simulink model "untitled"  (Simulink 8.5)
settings: Solver=ode45  StartTime=0.0  StopTime=0.04  FixedStep=0.0001  RelTol=1e-3
libraries: powerlib x131
settings Model: Creator=yahya  LastModifiedBy=yahya
settings DebuggingCC: SolverPrmCheckMsg=warning  FcnCallInpInsideContextMsg=EnableAllAsWarning
settings GRTTargetCC: CombineOutputUpdateFcns=on  GRTInterface=off

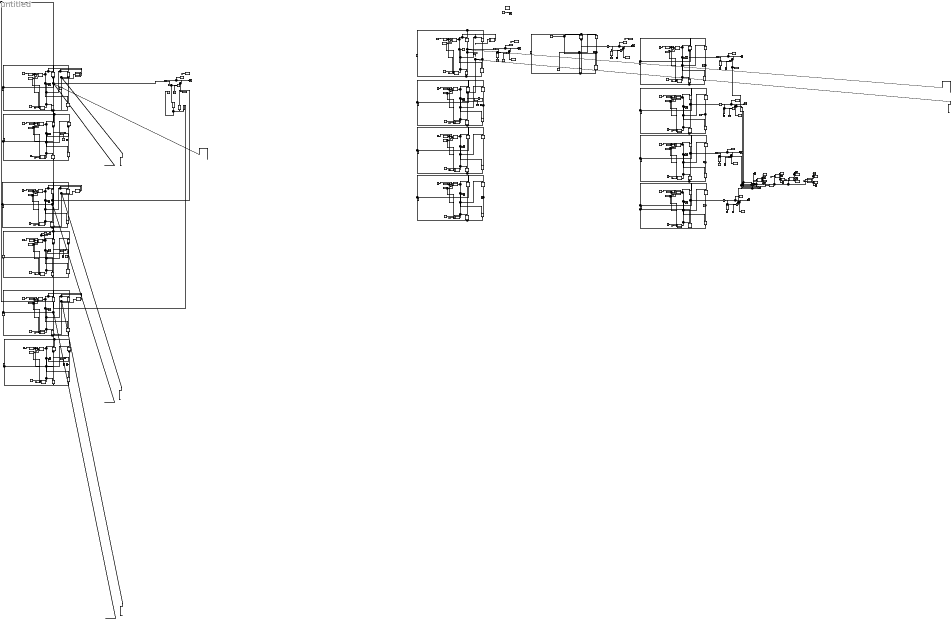
== system untitled ==
  Clock{,1..34} (35 alike) : Clock
  Current Measurement{,1..6} (7 alike) : powerlib/Measurements/Current Measurement  PhasorSimulation=off  OutputType=Complex  PSBequivalent=0
  DC Voltage Source{,1..14} (15 alike) : powerlib/Electrical Sources/DC Voltage Source  Amplitude=100  Measurements=None
  From Workspace1 : FromWorkspace  VariableName=tetha12  SampleTime=0
  From Workspace10 : FromWorkspace  VariableName=tetha11  SampleTime=0
  From Workspace{2,4,6,8,11..12,14,16,18,20,22,24,26,33} (14 alike) : FromWorkspace  VariableName=fs  SampleTime=0
  From Workspace13 : FromWorkspace  VariableName=tetha14  SampleTime=0
  From Workspace15 : FromWorkspace  VariableName=tetha12  SampleTime=0
  From Workspace17 : FromWorkspace  VariableName=tetha11  SampleTime=0
  From Workspace19 : FromWorkspace  VariableName=tetha12_120  SampleTime=0
  From Workspace21 : FromWorkspace  VariableName=tetha11_120  SampleTime=0
  From Workspace23 : FromWorkspace  VariableName=tetha12_240  SampleTime=0
  From Workspace25 : FromWorkspace  VariableName=tetha11_240  SampleTime=0
  From Workspace3 : FromWorkspace  VariableName=tetha13  SampleTime=0
  From Workspace32 : FromWorkspace  VariableName=tetha11  SampleTime=0
  From Workspace5 : FromWorkspace  VariableName=tetha14  SampleTime=0
  From Workspace7 : FromWorkspace  VariableName=tetha12  SampleTime=0
  From Workspace9 : FromWorkspace  VariableName=tetha13  SampleTime=0
  Ground{1..28} (28 alike) : powerlib/Elements/Ground  LConnTagsString=a
  IGBT/Diode{1..60} (60 alike) : powerlib/Power Electronics/IGBT//Diode  Ron=1e-3  Rs=1e5  Cs=inf  Measurements=off
  MATLAB Function : MATLAB Function  TreatAsAtomicUnit=on
  MATLAB Function1 : MATLAB Function  TreatAsAtomicUnit=on
  MATLAB Function10 : MATLAB Function  TreatAsAtomicUnit=on
  MATLAB Function11 : MATLAB Function  TreatAsAtomicUnit=on
  MATLAB Function12 : MATLAB Function  TreatAsAtomicUnit=on
  MATLAB Function13 : MATLAB Function  TreatAsAtomicUnit=on
  MATLAB Function14 : MATLAB Function  TreatAsAtomicUnit=on
  MATLAB Function15 : MATLAB Function  TreatAsAtomicUnit=on
  MATLAB Function16 : MATLAB Function  TreatAsAtomicUnit=on
  MATLAB Function17 : MATLAB Function  TreatAsAtomicUnit=on
  MATLAB Function18 : MATLAB Function  TreatAsAtomicUnit=on
  MATLAB Function19 : MATLAB Function  TreatAsAtomicUnit=on
  MATLAB Function2 : MATLAB Function  TreatAsAtomicUnit=on
  MATLAB Function20 : MATLAB Function  TreatAsAtomicUnit=on
  MATLAB Function21 : MATLAB Function  TreatAsAtomicUnit=on
  MATLAB Function22 : MATLAB Function  TreatAsAtomicUnit=on
  MATLAB Function23 : MATLAB Function  TreatAsAtomicUnit=on
  MATLAB Function24 : MATLAB Function  TreatAsAtomicUnit=on
  MATLAB Function25 : MATLAB Function  TreatAsAtomicUnit=on
  MATLAB Function26 : MATLAB Function  TreatAsAtomicUnit=on
  MATLAB Function27 : MATLAB Function  TreatAsAtomicUnit=on
  MATLAB Function28 : MATLAB Function  TreatAsAtomicUnit=on
  MATLAB Function29 : MATLAB Function  TreatAsAtomicUnit=on
  MATLAB Function3 : MATLAB Function  TreatAsAtomicUnit=on
  MATLAB Function30 : MATLAB Function  TreatAsAtomicUnit=on
  MATLAB Function31 : MATLAB Function  TreatAsAtomicUnit=on
  MATLAB Function32 : MATLAB Function  TreatAsAtomicUnit=on
  MATLAB Function33 : MATLAB Function  TreatAsAtomicUnit=on
  MATLAB Function34 : MATLAB Function  TreatAsAtomicUnit=on
  MATLAB Function35 : MATLAB Function  TreatAsAtomicUnit=on
  MATLAB Function4 : MATLAB Function  TreatAsAtomicUnit=on
  MATLAB Function5 : MATLAB Function  TreatAsAtomicUnit=on
  MATLAB Function6 : MATLAB Function  TreatAsAtomicUnit=on
  MATLAB Function7 : MATLAB Function  TreatAsAtomicUnit=on
  MATLAB Function8 : MATLAB Function  TreatAsAtomicUnit=on
  MATLAB Function9 : MATLAB Function  TreatAsAtomicUnit=on
  Pulse Generator{,2,5,7..8,11,13,15,17,19,21} (11 alike) : DiscretePulseGenerator  PulseType=Time based  Amplitude=10  Period=0.02  PulseWidth=50
  Pulse Generator{1,3,6,9..10,12,14,16,18,20,22} (11 alike) : DiscretePulseGenerator  PulseType=Time based  Amplitude=10  Period=0.02  PulseWidth=50  PhaseDelay=0.01
  Pulse Generator23 : DiscretePulseGenerator  PulseType=Time based  Amplitude=10  Period=0.02  PulseWidth=50  PhaseDelay=0.006666666666667
  Pulse Generator24 : DiscretePulseGenerator  PulseType=Time based  Amplitude=10  Period=0.02  PulseWidth=50  PhaseDelay=0.01+0.006666666666667
  Pulse Generator25 : DiscretePulseGenerator  PulseType=Time based  Amplitude=10  Period=0.02  PulseWidth=50  PhaseDelay=0.006666666666667
  Pulse Generator26 : DiscretePulseGenerator  PulseType=Time based  Amplitude=10  Period=0.02  PulseWidth=50  PhaseDelay=0.01+0.006666666666667
  Pulse Generator27 : DiscretePulseGenerator  PulseType=Time based  Amplitude=10  Period=0.02  PulseWidth=50  PhaseDelay=2*0.006666666666667
  Pulse Generator28 : DiscretePulseGenerator  PulseType=Time based  Amplitude=10  Period=0.02  PulseWidth=50  PhaseDelay=0.01+2*0.006666666666667
  Pulse Generator29 : DiscretePulseGenerator  PulseType=Time based  Amplitude=10  Period=0.02  PulseWidth=50  PhaseDelay=2*0.006666666666667
  Pulse Generator30 : DiscretePulseGenerator  PulseType=Time based  Amplitude=10  Period=0.02  PulseWidth=50  PhaseDelay=0.01+2*0.006666666666667
  Pulse Generator4 : DiscretePulseGenerator  PulseType=Time based  Period=0.0001  PulseWidth=50
  Scope{,1,4,6..14,25} (13 alike) : Scope  NumInputPorts=2
      Scope settings: TimeRange=1  YMin=-400~-400  YMax=400~400
      Scope1 settings: TimeRange=1  YMin=-400~-400  YMax=400~400
      Scope10 settings: TimeRange=1  YMin=-400~-400  YMax=400~400  SaveName=ScopeData4
      Scope11 settings: TimeRange=1  YMin=-400~-400  YMax=400~400  SaveName=ScopeData11
      Scope12 settings: TimeRange=1  YMin=-400~-400  YMax=400~400  SaveName=ScopeData12
      Scope13 settings: TimeRange=1  YMin=-400~-400  YMax=400~400  SaveName=ScopeData13
      Scope14 settings: TimeRange=1  YMin=-400~-400  YMax=400~400  SaveName=ScopeData14
      Scope25 settings: TimeRange=1  YMin=-400~-400  YMax=400~400  SaveName=ScopeData25
      Scope4 settings: TimeRange=1  YMin=-400~-400  YMax=400~400  SaveName=ScopeData6
      Scope6 settings: TimeRange=1  YMin=-400~-400  YMax=400~400  SaveName=ScopeData7
      Scope7 settings: TimeRange=1  YMin=-400~-400  YMax=400~400  SaveName=ScopeData9
      Scope8 settings: TimeRange=1  YMin=-400~-400  YMax=400~400  SaveName=ScopeData8
      Scope9 settings: TimeRange=1  YMin=-400~-400  YMax=400~400  SaveName=ScopeData10
  Scope15 : Scope  NumInputPorts=4
      settings: TimeRange=1  YMin=-400~-400~-5~-5  YMax=400~400~5~5  SaveName=ScopeData15
  Scope{16..24} (9 alike) : Scope
      Scope16 settings: TimeRange=0.2  YMin=190  YMax=400  SaveName=ScopeData16
      Scope17 settings: TimeRange=0.2  YMin=190  YMax=400  SaveName=ScopeData17
      Scope18 settings: TimeRange=0.2  YMin=190  YMax=400  SaveName=ScopeData18
      Scope19 settings: TimeRange=0.2  YMin=190  YMax=400  SaveName=ScopeData19
      Scope20 settings: TimeRange=0.2  YMin=190  YMax=400  SaveName=ScopeData20
      Scope21 settings: TimeRange=0.2  YMin=190  YMax=400  SaveName=ScopeData21
      Scope22 settings: TimeRange=0.2  YMin=190  YMax=400  SaveName=ScopeData22
      Scope23 settings: TimeRange=0.2  YMin=190  YMax=400  SaveName=ScopeData23
      Scope24 settings: TimeRange=0.2  YMin=190  YMax=400  SaveName=ScopeData24
  Scope{2..3,5,26..32} (10 alike) : Scope  NumInputPorts=3
      Scope2 settings: TimeRange=1  YMin=-400~-400~-5  YMax=400~400~5  SaveName=ScopeData3
      Scope26 settings: TimeRange=1  YMin=-400~-400~-5  YMax=400~400~5  SaveName=ScopeData26
      Scope27 settings: TimeRange=1  YMin=-400~-400~-5  YMax=400~400~5  SaveName=ScopeData27
      Scope28 settings: TimeRange=1  YMin=-400~-400~-5  YMax=400~400~5  SaveName=ScopeData28
      Scope29 settings: TimeRange=1  YMin=-400~-400~-5  YMax=400~400~5  SaveName=ScopeData29
      Scope3 settings: TimeRange=0.03572500664993174  YMin=-1~0~0  YMax=1~10~10  SaveName=ScopeData2
      Scope30 settings: TimeRange=1  YMin=-400~-400~-5  YMax=400~400~5  SaveName=ScopeData30
      Scope31 settings: TimeRange=1  YMin=-400~-400~-5  YMax=400~400~5  SaveName=ScopeData31
      Scope32 settings: TimeRange=1  YMin=-400~-400~-5  YMax=400~400~5  SaveName=ScopeData32
      Scope5 settings: TimeRange=1  YMin=-400~-400~-5  YMax=400~400~5  SaveName=ScopeData5
  Series RLC Branch{,6..8} (4 alike) : powerlib/Elements/Series RLC Branch  LConnTagsString=__new0  RConnTagsString=__new0  BranchType=R  Resistance=1  Inductance=1e-3  SetiL0=off  InitialCurrent=0  Capacitance=1e-6  Setx0=off  InitialVoltage=0  Measurements=None
  Series RLC Branch1 : powerlib/Elements/Series RLC Branch  LConnTagsString=__new0  RConnTagsString=__new0  BranchType=RL  Resistance=1  Inductance=1e-3  SetiL0=off  InitialCurrent=0  Capacitance=1e-6  Setx0=off  InitialVoltage=0  Measurements=None
  Series RLC Branch{2..5} (4 alike) : powerlib/Elements/Series RLC Branch  LConnTagsString=__new0  RConnTagsString=__new0  BranchType=R  Resistance=1  Inductance=1e-5  SetiL0=off  InitialCurrent=0  Capacitance=1e-6  Setx0=off  InitialVoltage=0  Measurements=None
  Sum : Sum  Inputs=|++++
  To Workspace : ToWorkspace  VariableName=i  SaveFormat=Timeseries  SampleTime=-1
  To Workspace1 : ToWorkspace  VariableName=v  SaveFormat=Timeseries  SampleTime=-1
  To Workspace10 : ToWorkspace  VariableName=v3  SaveFormat=Timeseries  SampleTime=-1
  To Workspace11 : ToWorkspace  VariableName=A1  SaveFormat=Timeseries  SampleTime=-1
  To Workspace12 : ToWorkspace  VariableName=i4  SaveFormat=Timeseries  SampleTime=-1
  To Workspace13 : ToWorkspace  VariableName=v4  SaveFormat=Timeseries  SampleTime=-1
  To Workspace14 : ToWorkspace  VariableName=B1  SaveFormat=Timeseries  SampleTime=-1
  To Workspace15 : ToWorkspace  VariableName=i5  SaveFormat=Timeseries  SampleTime=-1
  To Workspace16 : ToWorkspace  VariableName=v5  SaveFormat=Timeseries  SampleTime=-1
  To Workspace17 : ToWorkspace  VariableName=A7  SaveFormat=Timeseries  SampleTime=-1
  To Workspace18 : ToWorkspace  VariableName=B7  SaveFormat=Timeseries  SampleTime=-1
  To Workspace19 : ToWorkspace  VariableName=A11  SaveFormat=Timeseries  SampleTime=-1
  To Workspace2 : ToWorkspace  VariableName=t  SaveFormat=Timeseries  SampleTime=-1
  To Workspace20 : ToWorkspace  VariableName=B11  SaveFormat=Timeseries  SampleTime=-1
  To Workspace21 : ToWorkspace  VariableName=A5  SaveFormat=Timeseries  SampleTime=-1
  To Workspace22 : ToWorkspace  VariableName=B5  SaveFormat=Timeseries  SampleTime=-1
  To Workspace23 : ToWorkspace  VariableName=i6  SaveFormat=Timeseries  SampleTime=-1
  To Workspace24 : ToWorkspace  VariableName=v6  SaveFormat=Timeseries  SampleTime=-1
  To Workspace25 : ToWorkspace  VariableName=t2  SaveFormat=Timeseries  SampleTime=-1
  To Workspace3 : ToWorkspace  VariableName=i1  SaveFormat=Timeseries  SampleTime=-1
  To Workspace4 : ToWorkspace  VariableName=v1  SaveFormat=Timeseries  SampleTime=-1
  To Workspace5 : ToWorkspace  VariableName=t1  SaveFormat=Timeseries  SampleTime=-1
  To Workspace6 : ToWorkspace  VariableName=i2  SaveFormat=Timeseries  SampleTime=-1
  To Workspace7 : ToWorkspace  VariableName=v2  SaveFormat=Timeseries  SampleTime=-1
  To Workspace8 : ToWorkspace  VariableName=v_phase  SaveFormat=Timeseries  SampleTime=-1
  To Workspace9 : ToWorkspace  VariableName=i3  SaveFormat=Timeseries  SampleTime=-1
  Unit Delay : UnitDelay  SampleTime=0.01
  Voltage Measurement{,1..10} (11 alike) : powerlib/Measurements/Voltage Measurement  PhasorSimulation=off  OutputType=Complex  PSBequivalent=0
  powergui : powerlib/powergui  Priority=1  SimulationMode=Continuous  SolverType=Tustin/Backward Euler (TBE)  SampleTime=50e-6  frequency=60  SPID=off  DisableSnubberDevices=off  DisableRonSwitches=off  DisableVfSwitches=off  SwTol=0  DisplayEquations=off  Interpol=off  methode=off  Ts=100  FunctionMessages=off  echomessages=off  HookPort=off  EnableUseOfTLC=off  x0status=blocks  frequencyindice=0  Pbase=100e6  ErrMax=1e-4  Iterations=50  UnitsV=kV  UnitsW=MW  buscounter=0  RestoreLinks=warning  ResistiveCurrentMeasurement=off  Frange=[0:2:500]  Ylog=off  Xlog=on  ShowGrid=off  save=off  variable=ZData  structure=0  ZoomFFT=off  StartTime=0.0  cycles=1  DisplayStyle=1  fundamental=60  FreqAxis=off  MaxFrequency=1000  frequencyindicesteady=1  RmsSteady=1  display=off
  wires:
  Current Measurement/1 -> To Workspace/1, Scope/1
  Voltage Measurement/1 -> To Workspace1/1, Scope/2
  Clock/1 -> To Workspace2/1
  From Workspace32/1 -> MATLAB Function1/2(t), MATLAB Function/2(t)
  From Workspace33/1 -> MATLAB Function1/4(fs), MATLAB Function/4(fs)
  Clock1/1 -> MATLAB Function/3(time)
  Pulse Generator/1 -> MATLAB Function/1(u)
  Clock2/1 -> MATLAB Function1/3(time)
  Pulse Generator1/1 -> MATLAB Function1/1(u)
  Current Measurement1/1 -> To Workspace3/1, Scope1/1
  Voltage Measurement1/1 -> To Workspace4/1, Scope1/2
  Clock3/1 -> To Workspace5/1
  Pulse Generator3/1 -> IGBT/Diode6/1, IGBT/Diode7/1
  Pulse Generator2/1 -> IGBT/Diode8/1, IGBT/Diode5/1
  Pulse Generator4/1 -> Scope3/1
  MATLAB Function/1(y) -> MATLAB Function20/1(u1), IGBT/Diode1/1, IGBT/Diode4/1, Scope2/1
  MATLAB Function1/1(y) -> IGBT/Diode3/1, MATLAB Function20/2(u2), IGBT/Diode2/1, Scope2/2
  From Workspace1/1 -> MATLAB Function3/2(t), MATLAB Function2/2(t)
  From Workspace2/1 -> MATLAB Function3/4(fs), MATLAB Function2/4(fs)
  Clock5/1 -> MATLAB Function2/3(time)
  Pulse Generator5/1 -> MATLAB Function2/1(u)
  Clock6/1 -> MATLAB Function3/3(time)
  Pulse Generator6/1 -> MATLAB Function3/1(u)
  MATLAB Function2/1(y) -> IGBT/Diode9/1, IGBT/Diode12/1, Scope5/1
  MATLAB Function3/1(y) -> IGBT/Diode11/1, IGBT/Diode10/1, Scope5/2
  From Workspace3/1 -> MATLAB Function5/2(t), MATLAB Function4/2(t)
  From Workspace4/1 -> MATLAB Function5/4(fs), MATLAB Function4/4(fs)
  Clock8/1 -> MATLAB Function4/3(time)
  Pulse Generator8/1 -> MATLAB Function4/1(u)
  Clock9/1 -> MATLAB Function5/3(time)
  Pulse Generator9/1 -> MATLAB Function5/1(u)
  MATLAB Function4/1(y) -> IGBT/Diode13/1, IGBT/Diode16/1, Scope8/1
  MATLAB Function5/1(y) -> IGBT/Diode15/1, IGBT/Diode14/1, Scope8/2
  From Workspace5/1 -> MATLAB Function7/2(t), MATLAB Function6/2(t)
  From Workspace6/1 -> MATLAB Function7/4(fs), MATLAB Function6/4(fs)
  Clock11/1 -> MATLAB Function6/3(time)
  Pulse Generator11/1 -> MATLAB Function6/1(u)
  Clock12/1 -> MATLAB Function7/3(time)
  Pulse Generator12/1 -> MATLAB Function7/1(u)
  MATLAB Function6/1(y) -> IGBT/Diode17/1, IGBT/Diode20/1, Scope11/1
  MATLAB Function7/1(y) -> IGBT/Diode19/1, IGBT/Diode18/1, Scope11/2
  Current Measurement2/1 -> To Workspace6/1, Scope4/1
  Voltage Measurement2/1 -> Sum/1, Scope15/1, To Workspace7/1, Scope4/2
  From Workspace10/1 -> MATLAB Function9/2(t), MATLAB Function8/2(t)
  From Workspace11/1 -> MATLAB Function9/4(fs), MATLAB Function8/4(fs)
  Clock7/1 -> MATLAB Function8/3(time)
  Pulse Generator7/1 -> MATLAB Function8/1(u)
  Clock14/1 -> MATLAB Function9/3(time)
  Pulse Generator10/1 -> MATLAB Function9/1(u)
  MATLAB Function8/1(y) -> IGBT/Diode21/1, IGBT/Diode35/1, Scope7/1
  MATLAB Function9/1(y) -> IGBT/Diode34/1, IGBT/Diode32/1, Scope7/2
  From Workspace7/1 -> MATLAB Function11/2(t), MATLAB Function10/2(t)
  From Workspace8/1 -> MATLAB Function11/4(fs), MATLAB Function10/4(fs)
  Clock15/1 -> MATLAB Function10/3(time)
  Pulse Generator15/1 -> MATLAB Function10/1(u)
  Clock16/1 -> MATLAB Function11/3(time)
  Pulse Generator16/1 -> MATLAB Function11/1(u)
  MATLAB Function10/1(y) -> IGBT/Diode36/1, IGBT/Diode24/1, Scope9/1
  MATLAB Function11/1(y) -> IGBT/Diode23/1, IGBT/Diode22/1, Scope9/2
  From Workspace9/1 -> MATLAB Function13/2(t), MATLAB Function12/2(t)
  From Workspace12/1 -> MATLAB Function13/4(fs), MATLAB Function12/4(fs)
  Clock17/1 -> MATLAB Function12/3(time)
  Pulse Generator17/1 -> MATLAB Function12/1(u)
  Clock18/1 -> MATLAB Function13/3(time)
  Pulse Generator18/1 -> MATLAB Function13/1(u)
  MATLAB Function12/1(y) -> IGBT/Diode25/1, IGBT/Diode28/1, Scope10/1
  MATLAB Function13/1(y) -> IGBT/Diode27/1, IGBT/Diode26/1, Scope10/2
  From Workspace13/1 -> MATLAB Function15/2(t), MATLAB Function14/2(t)
  From Workspace14/1 -> MATLAB Function15/4(fs), MATLAB Function14/4(fs)
  Clock10/1 -> MATLAB Function14/3(time)
  Pulse Generator13/1 -> MATLAB Function14/1(u)
  Clock13/1 -> MATLAB Function15/3(time)
  Pulse Generator14/1 -> MATLAB Function15/1(u)
  MATLAB Function14/1(y) -> IGBT/Diode29/1, IGBT/Diode33/1, Scope6/1
  MATLAB Function15/1(y) -> IGBT/Diode31/1, IGBT/Diode30/1, Scope6/2
  Current Measurement3/1 -> To Workspace9/1, Scope12/1
  Voltage Measurement3/1 -> Sum/2, Scope15/2, Scope12/2, To Workspace10/1
  Current Measurement4/1 -> To Workspace12/1, Scope13/1
  Voltage Measurement4/1 -> Scope15/3, Sum/3, To Workspace13/1, Scope13/2
  Current Measurement5/1 -> To Workspace15/1, Scope14/1
  Voltage Measurement5/1 -> Sum/4, Scope15/4, To Workspace16/1, Scope14/2
  Clock4/1 -> MATLAB Function16/2(time)
  MATLAB Function16/1(A1) -> To Workspace11/1, Scope17/1
  MATLAB Function16/2(B1) -> Scope18/1, To Workspace14/1
  Clock19/1 -> MATLAB Function17/2(time)
  MATLAB Function17/1(A7) -> Scope16/1, To Workspace17/1
  MATLAB Function17/2(B7) -> To Workspace18/1, Scope19/1
  Sum/1 -> Scope24/1, MATLAB Function18/1(u), MATLAB Function17/1(u), MATLAB Function19/1(u), To Workspace8/1, MATLAB Function16/1(u)
  Clock20/1 -> MATLAB Function18/2(time)
  MATLAB Function18/1(A11) -> Scope20/1, To Workspace19/1
  MATLAB Function18/2(B11) -> Scope21/1, To Workspace20/1
  Clock21/1 -> MATLAB Function19/2(time)
  MATLAB Function19/1(A5) -> Scope22/1, To Workspace21/1
  MATLAB Function19/2(B5) -> Scope23/1, To Workspace22/1
  ? -> Scope2/3
  Voltage Measurement7/1 -> Scope5/3
  MATLAB Function20/1(y) -> ?
  Current Measurement6/1 -> Scope25/1, To Workspace23/1
  Voltage Measurement6/1 -> To Workspace24/1, Scope25/2
  Clock22/1 -> To Workspace25/1
  From Workspace17/1 -> MATLAB Function22/2(t), MATLAB Function21/2(t)
  From Workspace18/1 -> MATLAB Function22/4(fs), MATLAB Function21/4(fs)
  Clock23/1 -> MATLAB Function21/3(time)
  Pulse Generator19/1 -> MATLAB Function21/1(u)
  Clock24/1 -> MATLAB Function22/3(time)
  Pulse Generator20/1 -> MATLAB Function22/1(u)
  MATLAB Function21/1(y) -> MATLAB Function24/1(u1), IGBT/Diode37/1, IGBT/Diode43/1, Scope26/1
  MATLAB Function22/1(y) -> IGBT/Diode42/1, MATLAB Function24/2(u2), IGBT/Diode41/1, Scope26/2
  From Workspace15/1 -> MATLAB Function25/2(t), MATLAB Function23/2(t)
  From Workspace16/1 -> MATLAB Function25/4(fs), MATLAB Function23/4(fs)
  Clock25/1 -> MATLAB Function23/3(time)
  Pulse Generator21/1 -> MATLAB Function23/1(u)
  Clock26/1 -> MATLAB Function25/3(time)
  Pulse Generator22/1 -> MATLAB Function25/1(u)
  MATLAB Function23/1(y) -> IGBT/Diode44/1, IGBT/Diode40/1, Scope27/1
  MATLAB Function25/1(y) -> IGBT/Diode39/1, IGBT/Diode38/1, Scope27/2
  ? -> Scope26/3
  Voltage Measurement8/1 -> Scope27/3
  MATLAB Function24/1(y) -> ?
  From Workspace21/1 -> MATLAB Function27/2(t), MATLAB Function26/2(t)
  From Workspace22/1 -> MATLAB Function27/4(fs), MATLAB Function26/4(fs)
  Clock27/1 -> MATLAB Function26/3(time)
  Pulse Generator23/1 -> MATLAB Function26/1(u)
  Clock28/1 -> MATLAB Function27/3(time)
  Pulse Generator24/1 -> MATLAB Function27/1(u)
  MATLAB Function26/1(y) -> MATLAB Function29/1(u1), IGBT/Diode45/1, IGBT/Diode51/1, Scope28/1
  MATLAB Function27/1(y) -> IGBT/Diode50/1, MATLAB Function29/2(u2), IGBT/Diode49/1, Scope28/2
  From Workspace19/1 -> MATLAB Function30/2(t), MATLAB Function28/2(t)
  From Workspace20/1 -> MATLAB Function30/4(fs), MATLAB Function28/4(fs)
  Clock29/1 -> MATLAB Function28/3(time)
  Pulse Generator25/1 -> MATLAB Function28/1(u)
  Clock30/1 -> MATLAB Function30/3(time)
  Pulse Generator26/1 -> MATLAB Function30/1(u)
  MATLAB Function30/1(y) -> IGBT/Diode47/1, IGBT/Diode46/1, Scope29/2
  ? -> Scope28/3
  Voltage Measurement9/1 -> Scope29/3
  MATLAB Function29/1(y) -> ?
  From Workspace25/1 -> MATLAB Function32/2(t), MATLAB Function31/2(t)
  From Workspace26/1 -> MATLAB Function32/4(fs), MATLAB Function31/4(fs)
  Clock31/1 -> MATLAB Function31/3(time)
  Pulse Generator27/1 -> MATLAB Function31/1(u)
  Clock32/1 -> MATLAB Function32/3(time)
  Pulse Generator28/1 -> MATLAB Function32/1(u)
  MATLAB Function31/1(y) -> MATLAB Function34/1(u1), IGBT/Diode53/1, IGBT/Diode59/1, Scope30/1
  MATLAB Function32/1(y) -> IGBT/Diode58/1, MATLAB Function34/2(u2), IGBT/Diode57/1, Scope30/2
  From Workspace23/1 -> MATLAB Function35/2(t), MATLAB Function33/2(t)
  From Workspace24/1 -> MATLAB Function35/4(fs), MATLAB Function33/4(fs)
  Clock33/1 -> MATLAB Function33/3(time)
  Pulse Generator29/1 -> MATLAB Function33/1(u)
  Clock34/1 -> MATLAB Function35/3(time)
  Pulse Generator30/1 -> MATLAB Function35/1(u)
  MATLAB Function33/1(y) -> IGBT/Diode60/1, IGBT/Diode56/1, Scope31/1
  MATLAB Function35/1(y) -> IGBT/Diode55/1, IGBT/Diode54/1, Scope31/2
  ? -> Scope30/3
  Voltage Measurement10/1 -> Scope31/3
  MATLAB Function34/1(y) -> ?
  MATLAB Function28/1(y) -> Unit Delay/1, Scope32/3, IGBT/Diode52/1, IGBT/Diode48/1, Scope29/1
  Unit Delay/1 -> Scope32/1
  connections:
  IGBT/Diode2/LConn1 -- IGBT/Diode1/LConn1 -- DC Voltage Source/RConn1
  IGBT/Diode4/RConn1 -- DC Voltage Source/LConn1 -- IGBT/Diode3/RConn1
  Series RLC Branch/RConn1 -- Ground1/LConn1
  Current Measurement/RConn1 -- Voltage Measurement/LConn1 -- Series RLC Branch/LConn1
  Voltage Measurement/LConn2 -- Ground2/LConn1
  IGBT/Diode12/LConn1 -- Ground19/LConn1 -- IGBT/Diode10/RConn1
  IGBT/Diode7/RConn1 -- IGBT/Diode8/RConn1 -- DC Voltage Source1/LConn1
  Current Measurement1/RConn1 -- Voltage Measurement1/LConn1
  IGBT/Diode8/LConn1 -- Ground6/LConn1 -- IGBT/Diode6/RConn1
  IGBT/Diode5/RConn1 -- IGBT/Diode7/LConn1 -- Current Measurement1/LConn1
  Voltage Measurement1/LConn2 -- Ground5/LConn1
  IGBT/Diode6/LConn1 -- IGBT/Diode5/LConn1 -- DC Voltage Source1/RConn1
  Series RLC Branch1/RConn1 -- Ground4/LConn1
  DC Voltage Source2/RConn1 -- IGBT/Diode10/LConn1 -- IGBT/Diode9/LConn1
  IGBT/Diode11/RConn1 -- IGBT/Diode12/RConn1 -- DC Voltage Source2/LConn1
  DC Voltage Source3/RConn1 -- IGBT/Diode14/LConn1 -- IGBT/Diode13/LConn1
  IGBT/Diode15/RConn1 -- IGBT/Diode16/RConn1 -- DC Voltage Source3/LConn1
  IGBT/Diode15/LConn1 -- IGBT/Diode13/RConn1
  DC Voltage Source4/RConn1 -- IGBT/Diode18/LConn1 -- IGBT/Diode17/LConn1
  IGBT/Diode19/RConn1 -- IGBT/Diode20/RConn1 -- DC Voltage Source4/LConn1
  IGBT/Diode16/LConn1 -- IGBT/Diode14/RConn1
  IGBT/Diode20/LConn1 -- Ground3/LConn1 -- IGBT/Diode18/RConn1
  DC Voltage Source5/RConn1 -- IGBT/Diode32/LConn1 -- IGBT/Diode21/LConn1
  IGBT/Diode34/RConn1 -- IGBT/Diode35/RConn1 -- DC Voltage Source5/LConn1
  Series RLC Branch2/LConn1 -- Current Measurement2/RConn1 -- Voltage Measurement2/LConn1
  IGBT/Diode21/RConn1 -- IGBT/Diode34/LConn1 -- Current Measurement2/LConn1
  DC Voltage Source6/RConn1 -- IGBT/Diode22/LConn1 -- IGBT/Diode36/LConn1
  IGBT/Diode23/RConn1 -- IGBT/Diode24/RConn1 -- DC Voltage Source6/LConn1
  IGBT/Diode23/LConn1 -- Current Measurement3/LConn1 -- IGBT/Diode36/RConn1
  DC Voltage Source7/RConn1 -- IGBT/Diode26/LConn1 -- IGBT/Diode25/LConn1
  IGBT/Diode27/RConn1 -- IGBT/Diode28/RConn1 -- DC Voltage Source7/LConn1
  IGBT/Diode24/LConn1 -- Ground17/LConn1 -- IGBT/Diode22/RConn1
  DC Voltage Source8/RConn1 -- IGBT/Diode30/LConn1 -- IGBT/Diode29/LConn1
  DC Voltage Source8/LConn1 -- IGBT/Diode33/RConn1 -- IGBT/Diode31/RConn1
  IGBT/Diode28/LConn1 -- Ground16/LConn1 -- IGBT/Diode26/RConn1
  IGBT/Diode33/LConn1 -- Ground9/LConn1 -- IGBT/Diode30/RConn1
  Series RLC Branch2/RConn1 -- Ground7/LConn1
  Voltage Measurement2/LConn2 -- Ground8/LConn1
  IGBT/Diode35/LConn1 -- Ground18/LConn1 -- IGBT/Diode32/RConn1
  IGBT/Diode27/LConn1 -- IGBT/Diode25/RConn1 -- Current Measurement4/LConn1
  IGBT/Diode31/LConn1 -- Current Measurement5/LConn1 -- IGBT/Diode29/RConn1
  Series RLC Branch3/LConn1 -- Current Measurement3/RConn1 -- Voltage Measurement3/LConn1
  Series RLC Branch3/RConn1 -- Ground10/LConn1
  Voltage Measurement3/LConn2 -- Ground11/LConn1
  Series RLC Branch4/LConn1 -- Current Measurement4/RConn1 -- Voltage Measurement4/LConn1
  Series RLC Branch4/RConn1 -- Ground12/LConn1
  Voltage Measurement4/LConn2 -- Ground13/LConn1
  Series RLC Branch5/LConn1 -- Current Measurement5/RConn1 -- Voltage Measurement5/LConn1
  Series RLC Branch5/RConn1 -- Ground14/LConn1
  Voltage Measurement5/LConn2 -- Ground15/LConn1
  IGBT/Diode19/LConn1 -- IGBT/Diode17/RConn1
  ?
  Voltage Measurement7/LConn2 -- Ground21/LConn1
  IGBT/Diode3/LConn1 -- Current Measurement/LConn1 -- IGBT/Diode1/RConn1
  IGBT/Diode4/LConn1 -- IGBT/Diode9/RConn1 -- IGBT/Diode11/LConn1 -- Voltage Measurement7/LConn1 -- IGBT/Diode2/RConn1
  DC Voltage Source9/RConn1 -- IGBT/Diode41/LConn1 -- IGBT/Diode37/LConn1
  IGBT/Diode42/RConn1 -- IGBT/Diode43/RConn1 -- DC Voltage Source9/LConn1
  Series RLC Branch6/LConn1 -- Current Measurement6/RConn1 -- Voltage Measurement6/LConn1
  IGBT/Diode38/RConn1 -- IGBT/Diode40/LConn1 -- Ground22/LConn1
  IGBT/Diode44/LConn1 -- DC Voltage Source10/RConn1 -- IGBT/Diode38/LConn1
  DC Voltage Source10/LConn1 -- IGBT/Diode39/RConn1 -- IGBT/Diode40/RConn1
  IGBT/Diode37/RConn1 -- Current Measurement6/LConn1 -- IGBT/Diode42/LConn1
  IGBT/Diode41/RConn1 -- IGBT/Diode43/LConn1 -- IGBT/Diode44/RConn1 -- IGBT/Diode39/LConn1 -- Voltage Measurement8/LConn1
  ?
  Series RLC Branch6/RConn1 -- Series RLC Branch7/RConn1 -- Series RLC Branch8/RConn1 -- Ground20/LConn1
  Voltage Measurement6/LConn2 -- Ground23/LConn1
  Voltage Measurement8/LConn2 -- Ground24/LConn1
  DC Voltage Source12/RConn1 -- IGBT/Diode49/LConn1 -- IGBT/Diode45/LConn1
  IGBT/Diode50/RConn1 -- IGBT/Diode51/RConn1 -- DC Voltage Source12/LConn1
  IGBT/Diode46/RConn1 -- IGBT/Diode48/LConn1 -- Ground25/LConn1
  IGBT/Diode52/LConn1 -- DC Voltage Source11/RConn1 -- IGBT/Diode46/LConn1
  DC Voltage Source11/LConn1 -- IGBT/Diode47/RConn1 -- IGBT/Diode48/RConn1
  IGBT/Diode50/LConn1 -- Series RLC Branch7/LConn1 -- IGBT/Diode45/RConn1
  IGBT/Diode49/RConn1 -- IGBT/Diode51/LConn1 -- IGBT/Diode52/RConn1 -- IGBT/Diode47/LConn1 -- Voltage Measurement9/LConn1
  Voltage Measurement9/LConn2 -- Ground26/LConn1
  DC Voltage Source14/RConn1 -- IGBT/Diode57/LConn1 -- IGBT/Diode53/LConn1
  IGBT/Diode58/RConn1 -- IGBT/Diode59/RConn1 -- DC Voltage Source14/LConn1
  IGBT/Diode54/RConn1 -- IGBT/Diode56/LConn1 -- Ground27/LConn1
  IGBT/Diode60/LConn1 -- IGBT/Diode54/LConn1 -- DC Voltage Source13/RConn1
  DC Voltage Source13/LConn1 -- IGBT/Diode55/RConn1 -- IGBT/Diode56/RConn1
  IGBT/Diode58/LConn1 -- Series RLC Branch8/LConn1 -- IGBT/Diode53/RConn1
  IGBT/Diode57/RConn1 -- IGBT/Diode59/LConn1 -- IGBT/Diode55/LConn1 -- Voltage Measurement10/LConn1 -- IGBT/Diode60/RConn1
  Voltage Measurement10/LConn2 -- Ground28/LConn1

== matlab function MATLAB Function1 ==
  data: u input double; y output double; t input double; time input double; fs input double
function y = fcn(u,t,time,fs)
%#codegen
Q = fs/2;
z1 = mod(time,fs);
t1 = time-z1;
w = (t1/fs)+1;
fs = (fs*w);
z = (fs)-t;
t = t+fs-Q;
if t <= time && time <= z
    y = u;
else
    y = 0;
end
end

== matlab function MATLAB Function ==
  data: u input double; y output double; t input double; time input double; fs input double
function y = fcn(u,t,time,fs)
%#codegen
Q = fs;
z1 = mod(time,fs);
t1 = time-z1;
w = (t1/fs)+1;
fs = (fs*w)-(fs/2);
z = (fs)-t;
fs = fs-(Q/2);
t = t+fs;
if u > 0 && t <= time && time <= z
    y = u;
else
    y = 0;
end
end

== matlab function MATLAB Function2 ==
  data: u input double; y output double; t input double; time input double; fs input double
function y = fcn(u,t,time,fs)
%#codegen
Q = fs;
z1 = mod(time,fs);
t1 = time-z1;
w = (t1/fs)+1;
fs = (fs*w)-(fs/2);
z = (fs)-t;
fs = fs-(Q/2);
t = t+fs;
if u > 0 && t <= time && time <= z
    y = u;
else
    y = 0;
end
end

== matlab function MATLAB Function3 ==
  data: u input double; y output double; t input double; time input double; fs input double
function y = fcn(u,t,time,fs)
%#codegen
Q = fs/2;
z1 = mod(time,fs);
t1 = time-z1;
w = (t1/fs)+1;
fs = (fs*w);
z = (fs)-t;
t = t+fs-Q;
if t <= time && time <= z
    y = u;
else
    y = 0;
end
end

== matlab function MATLAB Function4 ==
  data: u input double; y output double; t input double; time input double; fs input double
function y = fcn(u,t,time,fs)
%#codegen
Q = fs;
z1 = mod(time,fs);
t1 = time-z1;
w = (t1/fs)+1;
fs = (fs*w)-(fs/2);
z = (fs)-t;
fs = fs-(Q/2);
t = t+fs;
if u > 0 && t <= time && time <= z
    y = u;
else
    y = 0;
end
end

== matlab function MATLAB Function5 ==
  data: u input double; y output double; t input double; time input double; fs input double
function y = fcn(u,t,time,fs)
%#codegen
Q = fs/2;
z1 = mod(time,fs);
t1 = time-z1;
w = (t1/fs)+1;
fs = (fs*w);
z = (fs)-t;
t = t+fs-Q;
if t <= time && time <= z
    y = u;
else
    y = 0;
end
end

== matlab function MATLAB Function6 ==
  data: u input double; y output double; t input double; time input double; fs input double
function y = fcn(u,t,time,fs)
%#codegen
Q = fs;
z1 = mod(time,fs);
t1 = time-z1;
w = (t1/fs)+1;
fs = (fs*w)-(fs/2);
z = (fs)-t;
fs = fs-(Q/2);
t = t+fs;
if u > 0 && t <= time && time <= z
    y = u;
else
    y = 0;
end
end

== matlab function MATLAB Function7 ==
  data: u input double; y output double; t input double; time input double; fs input double
function y = fcn(u,t,time,fs)
%#codegen
Q = fs/2;
z1 = mod(time,fs);
t1 = time-z1;
w = (t1/fs)+1;
fs = (fs*w);
z = (fs)-t;
t = t+fs-Q;
if t <= time && time <= z
    y = u;
else
    y = 0;
end
end

== matlab function MATLAB Function10 ==
  data: u input double; y output double; t input double; time input double; fs input double
function y = fcn(u,t,time,fs)
%#codegen
Q = fs;
z1 = mod(time,fs);
t1 = time-z1;
w = (t1/fs)+1;
fs = (fs*w)-(fs/2);
z = (fs)-t;
fs = fs-(Q/2);
t = t+fs;
if u > 0 && t <= time && time <= z
    y = u;
else
    y = 0;
end
end

== matlab function MATLAB Function11 ==
  data: u input double; y output double; t input double; time input double; fs input double
function y = fcn(u,t,time,fs)
%#codegen
Q = fs/2;
z1 = mod(time,fs);
t1 = time-z1;
w = (t1/fs)+1;
fs = (fs*w);
z = (fs)-t;
t = t+fs-Q;
if t <= time && time <= z
    y = u;
else
    y = 0;
end
end

== matlab function MATLAB Function12 ==
  data: u input double; y output double; t input double; time input double; fs input double
function y = fcn(u,t,time,fs)
%#codegen
Q = fs;
z1 = mod(time,fs);
t1 = time-z1;
w = (t1/fs)+1;
fs = (fs*w)-(fs/2);
z = (fs)-t;
fs = fs-(Q/2);
t = t+fs;
if u > 0 && t <= time && time <= z
    y = u;
else
    y = 0;
end
end

== matlab function MATLAB Function13 ==
  data: u input double; y output double; t input double; time input double; fs input double
function y = fcn(u,t,time,fs)
%#codegen
Q = fs/2;
z1 = mod(time,fs);
t1 = time-z1;
w = (t1/fs)+1;
fs = (fs*w);
z = (fs)-t;
t = t+fs-Q;
if t <= time && time <= z
    y = u;
else
    y = 0;
end
end

== matlab function MATLAB Function14 ==
  data: u input double; y output double; t input double; time input double; fs input double
function y = fcn(u,t,time,fs)
%#codegen
Q = fs;
z1 = mod(time,fs);
t1 = time-z1;
w = (t1/fs)+1;
fs = (fs*w)-(fs/2);
z = (fs)-t;
fs = fs-(Q/2);
t = t+fs;
if u > 0 && t <= time && time <= z
    y = u;
else
    y = 0;
end
end

== matlab function MATLAB Function15 ==
  data: u input double; y output double; t input double; time input double; fs input double
function y = fcn(u,t,time,fs)
%#codegen
Q = fs/2;
z1 = mod(time,fs);
t1 = time-z1;
w = (t1/fs)+1;
fs = (fs*w);
z = (fs)-t;
t = t+fs-Q;
if t <= time && time <= z
    y = u;
else
    y = 0;
end
end

== matlab function MATLAB Function8 ==
  data: u input double; y output double; t input double; time input double; fs input double
function y = fcn(u,t,time,fs)
%#codegen
Q = fs;
z1 = mod(time,fs);
t1 = time-z1;
w = (t1/fs)+1;
fs = (fs*w)-(fs/2);
z = (fs)-t;
fs = fs-(Q/2);
t = t+fs;
if u > 0 && t <= time && time <= z
    y = u;
else
    y = 0;
end
end

== matlab function MATLAB Function9 ==
  data: u input double; y output double; t input double; time input double; fs input double
function y = fcn(u,t,time,fs)
%#codegen
Q = fs/2;
z1 = mod(time,fs);
t1 = time-z1;
w = (t1/fs)+1;
fs = (fs*w);
z = (fs)-t;
t = t+fs-Q;
if t <= time && time <= z
    y = u;
else
    y = 0;
end
end

== matlab function MATLAB Function16 ==
  data: u input double; A1 output double; time input double; B1 output double
function [A1,B1] = fcn(u,time)
%#codegen
A1 = u*sin(2*pi*50*time);
B1 = u*cos(2*pi*50*time);
end

== matlab function MATLAB Function17 ==
  data: u input double; A7 output double; time input double; B7 output double
function [A7,B7] = fcn(u,time)
%#codegen
A7 = u*sin(7*2*pi*50*time);
B7 = u*cos(7*2*pi*50*time);
end

== matlab function MATLAB Function18 ==
  data: u input double; A11 output double; time input double; B11 output double
function [A11,B11] = fcn(u,time)
%#codegen
A11 = u*sin(11*2*pi*50*time);
B11 = u*cos(11*2*pi*50*time);
end

== matlab function MATLAB Function19 ==
  data: u input double; A5 output double; time input double; B5 output double
function [A5,B5] = fcn(u,time)
%#codegen
A5 = u*sin(5*2*pi*50*time);
B5 = u*cos(5*2*pi*50*time);
end

== matlab function MATLAB Function20 ==
  data: u1 input double; y output double; u2 input double
function y = fcn(u1,u2)
%#codegen
if u1 == 0 && u2 == 0
    y = 10 ;
else
    y = 0;
end

== matlab function MATLAB Function21 ==
  data: u input double; y output double; t input double; time input double; fs input double
function y = fcn(u,t,time,fs)
%#codegen
Q = fs;
z1 = mod(time,fs);
t1 = time-z1;
w = (t1/fs)+1;
fs = (fs*w)-(fs/2);
z = (fs)-t;
fs = fs-(Q/2);
t = t+fs;
if u > 0 && t <= time && time <= z
    y = u;
else
    y = 0;
end
end

== matlab function MATLAB Function22 ==
  data: u input double; y output double; t input double; time input double; fs input double
function y = fcn(u,t,time,fs)
%#codegen
Q = fs/2;
z1 = mod(time,fs);
t1 = time-z1;
w = (t1/fs)+1;
fs = (fs*w);
z = (fs)-t;
t = t+fs-Q;
if t <= time && time <= z
    y = u;
else
    y = 0;
end
end

== matlab function MATLAB Function23 ==
  data: u input double; y output double; t input double; time input double; fs input double
function y = fcn(u,t,time,fs)
%#codegen
Q = fs;
z1 = mod(time,fs);
t1 = time-z1;
w = (t1/fs)+1;
fs = (fs*w)-(fs/2);
z = (fs)-t;
fs = fs-(Q/2);
t = t+fs;
if u > 0 && t <= time && time <= z
    y = u;
else
    y = 0;
end
end

== matlab function MATLAB Function24 ==
  data: u1 input double; y output double; u2 input double
function y = fcn(u1,u2)
%#codegen
if u1 == 0 && u2 == 0
    y = 10 ;
else
    y = 0;
end

== matlab function MATLAB Function25 ==
  data: u input double; y output double; t input double; time input double; fs input double
function y = fcn(u,t,time,fs)
%#codegen
Q = fs/2;
z1 = mod(time,fs);
t1 = time-z1;
w = (t1/fs)+1;
fs = (fs*w);
z = (fs)-t;
t = t+fs-Q;
if t <= time && time <= z
    y = u;
else
    y = 0;
end
end

== matlab function MATLAB Function26 ==
  data: u input double; y output double; t input double; time input double; fs input double
function y = fcn(u,t,time,fs)
%#codegen
Q = fs;
z1 = mod(time,fs);
t1 = time-z1;
w = (t1/fs)+1;
fs = (fs*w)-(fs/2);
z = (fs)-t;
fs = fs-(Q/2);
t = t+fs;
if u > 0 && t <= time && time <= z
    y = u;
else
    y = 0;
end
end

== matlab function MATLAB Function27 ==
  data: u input double; y output double; t input double; time input double; fs input double
function y = fcn(u,t,time,fs)
%#codegen
Q = fs/2;
z1 = mod(time,fs);
t1 = time-z1;
w = (t1/fs)+1;
fs = (fs*w);
z = (fs)-t;
t = t+fs-Q;
if t <= time && time <= z
    y = u;
else
    y = 0;
end
end

== matlab function MATLAB Function28 ==
  data: u input double; y output double; t input double; time input double; fs input double
function y = fcn(u,t,time,fs)
%#codegen
Q = fs;
z1 = mod(time,fs);
t1 = time-z1;
w = (t1/fs)+1;
fs = (fs*w)-(fs/2);
z = (fs)-t;
fs = fs-(Q/2);
t = t+fs;
if u > 0 && t <= time && time <= z
    y = u;
else
    y = 0;
end
end

== matlab function MATLAB Function29 ==
  data: u1 input double; y output double; u2 input double
function y = fcn(u1,u2)
%#codegen
if u1 == 0 && u2 == 0
    y = 10 ;
else
    y = 0;
end

== matlab function MATLAB Function30 ==
  data: u input double; y output double; t input double; time input double; fs input double
function y = fcn(u,t,time,fs)
%#codegen
Q = fs/2;
z1 = mod(time,fs);
t1 = time-z1;
w = (t1/fs)+1;
fs = (fs*w);
z = (fs)-t;
t = t+fs-Q;
if t <= time && time <= z
    y = u;
else
    y = 0;
end
end

== matlab function MATLAB Function31 ==
  data: u input double; y output double; t input double; time input double; fs input double
function y = fcn(u,t,time,fs)
%#codegen
Q = fs;
z1 = mod(time,fs);
t1 = time-z1;
w = (t1/fs)+1;
fs = (fs*w)-(fs/2);
z = (fs)-t;
fs = fs-(Q/2);
t = t+fs;
if u > 0 && t <= time && time <= z
    y = u;
else
    y = 0;
end
end

== matlab function MATLAB Function32 ==
  data: u input double; y output double; t input double; time input double; fs input double
function y = fcn(u,t,time,fs)
%#codegen
Q = fs/2;
z1 = mod(time,fs);
t1 = time-z1;
w = (t1/fs)+1;
fs = (fs*w);
z = (fs)-t;
t = t+fs-Q;
if t <= time && time <= z
    y = u;
else
    y = 0;
end
end

== matlab function MATLAB Function33 ==
  data: u input double; y output double; t input double; time input double; fs input double
function y = fcn(u,t,time,fs)
%#codegen
Q = fs;
z1 = mod(time,fs);
t1 = time-z1;
w = (t1/fs)+1;
fs = (fs*w)-(fs/2);
z = (fs)-t;
fs = fs-(Q/2);
t = t+fs;
if u > 0 && t <= time && time <= z
    y = u;
else
    y = 0;
end
end

== matlab function MATLAB Function34 ==
  data: u1 input double; y output double; u2 input double
function y = fcn(u1,u2)
%#codegen
if u1 == 0 && u2 == 0
    y = 10 ;
else
    y = 0;
end

== matlab function MATLAB Function35 ==
  data: u input double; y output double; t input double; time input double; fs input double
function y = fcn(u,t,time,fs)
%#codegen
Q = fs/2;
z1 = mod(time,fs);
t1 = time-z1;
w = (t1/fs)+1;
fs = (fs*w);
z = (fs)-t;
t = t+fs-Q;
if t <= time && time <= z
    y = u;
else
    y = 0;
end
end
